simulink model "untitled"  (R2020a)
settings: Solver=VariableStepAuto  StartTime=0.0  StopTime=10.0  RelTol=1e-3
settings Model: Creator=bill2  LastModifiedBy=bill2

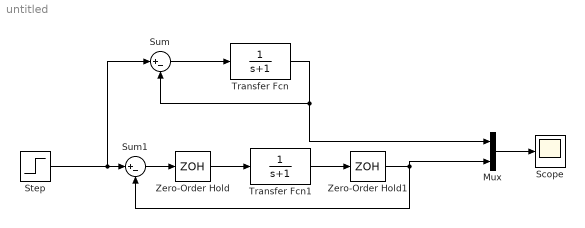
== system untitled ==
  Mux : Mux  Inputs=2
  Scope : Scope
  Step : Step  SampleTime=0
  Sum : Sum  Inputs=|+-
  Sum1 : Sum  Inputs=|+-
  Transfer Fcn : TransferFcn  Denominator=[1 1]
  Transfer Fcn1 : TransferFcn  Denominator=[1 1]
  Zero-Order Hold : ZeroOrderHold  SampleTime=-1
  Zero-Order Hold1 : ZeroOrderHold  SampleTime=-1
  wires:
  Step/1 -> Sum/1, Sum1/1
  Sum/1 -> Transfer Fcn/1
  Transfer Fcn/1 -> Mux/1, Sum/2
  Transfer Fcn1/1 -> Zero-Order Hold1/1
  Zero-Order Hold/1 -> Transfer Fcn1/1
  Sum1/1 -> Zero-Order Hold/1
  Zero-Order Hold1/1 -> Sum1/2, Mux/2
  Mux/1 -> Scope/1
